simulink model "task3_lab9"  (R2021a)
settings: Solver=FixedStepDiscrete  StartTime=0.0  StopTime=10.0  RelTol=1e-3
settings Model: Creator=reemb  LastModifiedBy=reemb
settings OptimizationCC: DefaultParameterBehavior=Inlined  EnhancedBackFolding=on  PassReuseOutputArgsAs=Individual arguments  ZeroExternalMemoryAtStartup=off  ZeroInternalMemoryAtStartup=off  OptimizeBlockOrder=speed  DifferentSizesBufferReuse=on  OptimizationCustomize=off  EfficientTunableParamExpr=on
settings DebuggingCC: ParameterTunabilityLossMsg=error
settings SFSimCC: MATLABDynamicMemAlloc=off
settings RTWCC: SystemTargetFile=ert.tlc  GenCodeOnly=on  TemplateMakefile=ert_default_tmf
settings CodeAppCC: ForceParamTrailComments=on  IgnoreCustomStorageClasses=off  OperatorAnnotations=on  SimulinkDataObjDesc=on  SFDataObjDesc=on  InsertBlockDesc=on
settings ERTTargetCC: TargetLangStandard=C99 (ISO)  GenerateSampleERTMain=on  InlinedParameterPlacement=NonHierarchical  ERTCustomFileTemplate=example_file_process.tlc

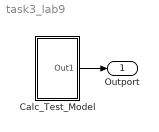
== system task3_lab9 ==
  Calc_Test_Model : Subsystem  TreatAsAtomicUnit=on  RTWFcnName=calc_functions
      settings: RTWFcnNameOpts=User specified  RTWFileNameOpts=Use function name
  Outport : Outport
  wires:
  Calc_Test_Model/1(Out1) -> Outport/1

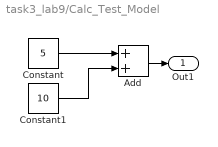
== system task3_lab9/Calc_Test_Model ==
  Add : Sum
  Constant : Constant  Value=5
  Constant1 : Constant  Value=10
  Out1 : Outport
  wires:
  Constant1/1 -> Add/2
  Constant/1 -> Add/1
  Add/1 -> Out1/1
